simulink model "Mmc"  (R2024b)
settings: Solver=ode23t  StartTime=0.0  StopTime=2  FixedStep=Ts_Power
values from neighbouring files (symbols this model uses):
  C_PM = 10e-3    (= 0.01)    [MmcParameters.m]
  eta = delta_wmax*(Vmax^2)/P_rated    (= 3.64590094798)    [MmcParameters.m]
  Fnom = 50    [MmcParameters.m]
  fs = 1000    [MmcParameters.m]
  I_b = Snom/Vnom_AC/sqrt(3)    [MmcParameters.m]
  Ipp_b = Snom/Vnom_AC/sqrt(3/2)    [MmcParameters.m]
  kicir = R0*alpha_ic    (= 523.598775598)    [MmcParameters.m]
  kpcir = L0*alpha_ic    (= 400)    [MmcParameters.m]
  L0 = 1.2 * L_b    (= 0.0763943726841)    [MmcParameters.m]
  mu = 2*eta*Q_rated/(N*((2*Vmax^2-V0^2)^2-V0^4))    [MmcParameters.m]
  Nb_PM = 20    [MmcParameters.m]
  phi_r = pi/2    (= 1.57079632679)    [MmcParameters.m]
  R0 = .1    (= 0.1)    [MmcParameters.m]
  SCR = 10    [MmcParameters.m]
  SigmaM = 10    [MmcParameters.m]
  Snom = 80e6    (= 80000000)    [MmcParameters.m]
  Ts_Power = 1e-5    (= 1e-05)    [MmcParameters.m]
  V0 = 1    [MmcParameters.m]
  V_b = Vnom_AC    (= 40000)    [MmcParameters.m]
  VDCm = 48e3    (= 48000)    [MmcParameters.m]
  VDCp = 48e3    (= 48000)    [MmcParameters.m]
  Vnom_AC = 40e3    (= 40000)    [MmcParameters.m]
  Vnom_PM = 4.8e3    (= 4800)    [MmcParameters.m]
  w_b = 2*pi*Fnom    (= 314.159265359)    [MmcParameters.m]
  Zn = Vnom_AC^2 / Snom    (= 20)    [MmcParameters.m]
undefined symbols (not defined in the file or in its folder): DiscIntNeverNeededParam
libraries: spsCurrentMeasurementLib x7, spsFirstOrderFilterLib x6, spsHalfBridgeMMCLib x6, spsSeriesRLCBranchLib x6, eePwmGeneratorMultilevel x6, spsVoltageMeasurementLib x4, spsGroundLib x2, spsMeanLib x2, spsDCVoltageSourceLib x2, spsThreePhaseVIMeasurementLib x2, slpidlib x2, spsThreePhaseSeriesRLCLoadLib x2
(part 2 of 3)

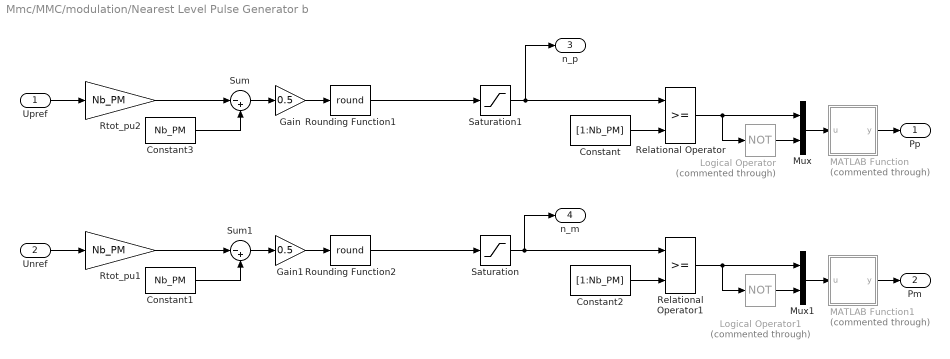
== system Mmc/MMC/modulation/Nearest Level Pulse Generator b ==
  Upref : Inport
  Unref : Inport  Port=2
  Constant : Constant  Value=[1:Nb_PM]
  Constant1 : Constant  Value=Nb_PM
  Constant2 : Constant  Value=[1:Nb_PM]
  Constant3 : Constant  Value=Nb_PM
  Gain : Gain  Gain=0.5
  Gain1 : Gain  Gain=0.5
  Logical Operator : Logic  Commented=through  Operator=NOT  AllPortsSameDT=off  OutDataTypeStr=float('double')
  Logical Operator1 : Logic  Commented=through  Operator=NOT  AllPortsSameDT=off  OutDataTypeStr=float('double')
  MATLAB Function : MATLAB Function  Commented=through  TreatAsAtomicUnit=on
  MATLAB Function1 : MATLAB Function  Commented=through  TreatAsAtomicUnit=on
  Mux : Mux  Inputs=2
  Mux1 : Mux  Inputs=2
  Relational Operator : RelationalOperator  OutDataTypeStr=float('double')  InputSameDT=off
  Relational Operator1 : RelationalOperator  OutDataTypeStr=float('double')  InputSameDT=off
  Rounding Function1 : Rounding  Operator=round
  Rounding Function2 : Rounding  Operator=round
  Rtot_pu1 : Gain  Gain=Nb_PM  SaturateOnIntegerOverflow=on  OutDataTypeStr=Inherit: Same as input  ParamDataTypeStr=Inherit: Same as input
  Rtot_pu2 : Gain  Gain=Nb_PM  SaturateOnIntegerOverflow=on  OutDataTypeStr=Inherit: Same as input  ParamDataTypeStr=Inherit: Same as input
  Saturation : Saturate  UpperLimit=Nb_PM  LowerLimit=0
  Saturation1 : Saturate  UpperLimit=Nb_PM  LowerLimit=0
  Sum : Sum  Inputs=|-+
  Sum1 : Sum  Inputs=|-+
  Pp : Outport  VectorParamsAs1DForOutWhenUnconnected=off
  Pm : Outport  Port=2  VectorParamsAs1DForOutWhenUnconnected=off
  n_p : Outport  Port=3  VectorParamsAs1DForOutWhenUnconnected=off
  n_m : Outport  Port=4  VectorParamsAs1DForOutWhenUnconnected=off
  wires:
  Gain1/1 -> Rounding Function2/1
  Constant1/1 -> Sum1/2
  Rtot_pu1/1 -> Sum1/1
  Unref/1 -> Rtot_pu1/1
  Sum1/1 -> Gain1/1
  Rounding Function2/1 -> Saturation/1
  Rounding Function1/1 -> Saturation1/1
  Saturation/1 -> Relational Operator1/1, n_m/1
  MATLAB Function1/1(y) -> Pm/1
  Mux1/1 -> MATLAB Function1/1(u)
  Logical Operator1/1 -> Mux1/2
  Relational Operator1/1 -> Logical Operator1/1, Mux1/1
  Constant2/1 -> Relational Operator1/2
  Upref/1 -> Rtot_pu2/1
  Gain/1 -> Rounding Function1/1
  Sum/1 -> Gain/1
  Constant3/1 -> Sum/2
  Rtot_pu2/1 -> Sum/1
  Saturation1/1 -> Relational Operator/1, n_p/1
  MATLAB Function/1(y) -> Pp/1
  Mux/1 -> MATLAB Function/1(u)
  Logical Operator/1 -> Mux/2
  Relational Operator/1 -> Mux/1, Logical Operator/1
  Constant/1 -> Relational Operator/2

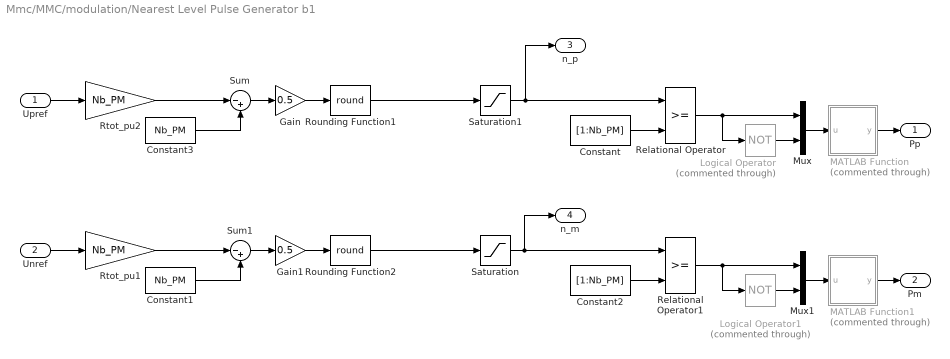
== system Mmc/MMC/modulation/Nearest Level Pulse Generator b1 ==
  Upref : Inport
  Unref : Inport  Port=2
  Constant : Constant  Value=[1:Nb_PM]
  Constant1 : Constant  Value=Nb_PM
  Constant2 : Constant  Value=[1:Nb_PM]
  Constant3 : Constant  Value=Nb_PM
  Gain : Gain  Gain=0.5
  Gain1 : Gain  Gain=0.5
  Logical Operator : Logic  Commented=through  Operator=NOT  AllPortsSameDT=off  OutDataTypeStr=float('double')
  Logical Operator1 : Logic  Commented=through  Operator=NOT  AllPortsSameDT=off  OutDataTypeStr=float('double')
  MATLAB Function : MATLAB Function  Commented=through  TreatAsAtomicUnit=on
  MATLAB Function1 : MATLAB Function  Commented=through  TreatAsAtomicUnit=on
  Mux : Mux  Inputs=2
  Mux1 : Mux  Inputs=2
  Relational Operator : RelationalOperator  OutDataTypeStr=float('double')  InputSameDT=off
  Relational Operator1 : RelationalOperator  OutDataTypeStr=float('double')  InputSameDT=off
  Rounding Function1 : Rounding  Operator=round
  Rounding Function2 : Rounding  Operator=round
  Rtot_pu1 : Gain  Gain=Nb_PM  SaturateOnIntegerOverflow=on  OutDataTypeStr=Inherit: Same as input  ParamDataTypeStr=Inherit: Same as input
  Rtot_pu2 : Gain  Gain=Nb_PM  SaturateOnIntegerOverflow=on  OutDataTypeStr=Inherit: Same as input  ParamDataTypeStr=Inherit: Same as input
  Saturation : Saturate  UpperLimit=Nb_PM  LowerLimit=0
  Saturation1 : Saturate  UpperLimit=Nb_PM  LowerLimit=0
  Sum : Sum  Inputs=|-+
  Sum1 : Sum  Inputs=|-+
  Pp : Outport  VectorParamsAs1DForOutWhenUnconnected=off
  Pm : Outport  Port=2  VectorParamsAs1DForOutWhenUnconnected=off
  n_p : Outport  Port=3  VectorParamsAs1DForOutWhenUnconnected=off
  n_m : Outport  Port=4  VectorParamsAs1DForOutWhenUnconnected=off
  wires:
  Gain1/1 -> Rounding Function2/1
  Constant1/1 -> Sum1/2
  Rtot_pu1/1 -> Sum1/1
  Unref/1 -> Rtot_pu1/1
  Sum1/1 -> Gain1/1
  Rounding Function2/1 -> Saturation/1
  Rounding Function1/1 -> Saturation1/1
  Saturation/1 -> Relational Operator1/1, n_m/1
  MATLAB Function1/1(y) -> Pm/1
  Mux1/1 -> MATLAB Function1/1(u)
  Logical Operator1/1 -> Mux1/2
  Relational Operator1/1 -> Logical Operator1/1, Mux1/1
  Constant2/1 -> Relational Operator1/2
  Upref/1 -> Rtot_pu2/1
  Gain/1 -> Rounding Function1/1
  Sum/1 -> Gain/1
  Constant3/1 -> Sum/2
  Rtot_pu2/1 -> Sum/1
  Saturation1/1 -> Relational Operator/1, n_p/1
  MATLAB Function/1(y) -> Pp/1
  Mux/1 -> MATLAB Function/1(u)
  Logical Operator/1 -> Mux/2
  Relational Operator/1 -> Mux/1, Logical Operator/1
  Constant/1 -> Relational Operator/2

== system Mmc/MMC/modulation/Sorting na ==
  note: A secrect, unintelligible, confusing and insrutable function with \if inside \for inside \if inside \if inside \if
  Usm : Inport
  N : Inport  Port=2
  Iarm : Inport  Port=3
  Constant : Constant  Value=SigmaM
  Logical Operator : Logic  Operator=NOT  AllPortsSameDT=off  OutDataTypeStr=float('double')
  MATLAB Function : MATLAB Function  TreatAsAtomicUnit=on
  MATLAB Function1 : MATLAB Function  TreatAsAtomicUnit=on
  Memory : Memory  InitialCondition=logical(zeros(Nb_PM, 1))  InheritSampleTime=on
  Mux : Mux  Inputs=2
  firing : Outport
  wires:
  MATLAB Function1/1(y) -> firing/1
  Logical Operator/1 -> Mux/2
  MATLAB Function/1(Ons_next) -> Mux/1, Logical Operator/1, Memory/1
  Mux/1 -> MATLAB Function1/1(u)
  Usm/1 -> MATLAB Function/1(Usm)
  Constant/1 -> MATLAB Function/3(Sigmam)
  N/1 -> MATLAB Function/2(N)
  Memory/1 -> MATLAB Function/5(Ons)
  Iarm/1 -> MATLAB Function/4(Iarm)

== system Mmc/MMC/modulation/Sorting nb ==
  note: A secrect, unintelligible, confusing and insrutable function with \if inside \for inside \if inside \if inside \if
  Usm : Inport
  N : Inport  Port=2
  Iarm : Inport  Port=3
  Constant : Constant  Value=SigmaM
  Logical Operator : Logic  Operator=NOT  AllPortsSameDT=off  OutDataTypeStr=float('double')
  MATLAB Function : MATLAB Function  TreatAsAtomicUnit=on
  MATLAB Function1 : MATLAB Function  TreatAsAtomicUnit=on
  Memory : Memory  InitialCondition=logical(zeros(Nb_PM, 1))  InheritSampleTime=on
  Mux : Mux  Inputs=2
  firing : Outport
  wires:
  MATLAB Function1/1(y) -> firing/1
  Logical Operator/1 -> Mux/2
  MATLAB Function/1(Ons_next) -> Mux/1, Logical Operator/1, Memory/1
  Mux/1 -> MATLAB Function1/1(u)
  Usm/1 -> MATLAB Function/1(Usm)
  Constant/1 -> MATLAB Function/3(Sigmam)
  N/1 -> MATLAB Function/2(N)
  Memory/1 -> MATLAB Function/5(Ons)
  Iarm/1 -> MATLAB Function/4(Iarm)

== system Mmc/MMC/modulation/Sorting nc ==
  note: A secrect, unintelligible, confusing and insrutable function with \if inside \for inside \if inside \if inside \if
  Usm : Inport
  N : Inport  Port=2
  Iarm : Inport  Port=3
  Constant : Constant  Value=SigmaM
  Logical Operator : Logic  Operator=NOT  AllPortsSameDT=off  OutDataTypeStr=float('double')
  MATLAB Function : MATLAB Function  TreatAsAtomicUnit=on
  MATLAB Function1 : MATLAB Function  TreatAsAtomicUnit=on
  Memory : Memory  InitialCondition=logical(zeros(Nb_PM, 1))  InheritSampleTime=on
  Mux : Mux  Inputs=2
  firing : Outport
  wires:
  MATLAB Function1/1(y) -> firing/1
  Logical Operator/1 -> Mux/2
  MATLAB Function/1(Ons_next) -> Mux/1, Logical Operator/1, Memory/1
  Mux/1 -> MATLAB Function1/1(u)
  Usm/1 -> MATLAB Function/1(Usm)
  Constant/1 -> MATLAB Function/3(Sigmam)
  N/1 -> MATLAB Function/2(N)
  Memory/1 -> MATLAB Function/5(Ons)
  Iarm/1 -> MATLAB Function/4(Iarm)

== system Mmc/MMC/modulation/Sorting pa ==
  note: A secrect, unintelligible, confusing and insrutable function with \if inside \for inside \if inside \if inside \if
  Usm : Inport
  N : Inport  Port=2
  Iarm : Inport  Port=3
  Constant : Constant  Value=SigmaM
  Logical Operator : Logic  Operator=NOT  AllPortsSameDT=off  OutDataTypeStr=float('double')
  MATLAB Function : MATLAB Function  TreatAsAtomicUnit=on
  MATLAB Function1 : MATLAB Function  TreatAsAtomicUnit=on
  Memory : Memory  InitialCondition=logical(zeros(Nb_PM, 1))  InheritSampleTime=on
  Mux : Mux  Inputs=2
  firing : Outport
  wires:
  Iarm/1 -> MATLAB Function/4(Iarm)
  Memory/1 -> MATLAB Function/5(Ons)
  N/1 -> MATLAB Function/2(N)
  Constant/1 -> MATLAB Function/3(Sigmam)
  Usm/1 -> MATLAB Function/1(Usm)
  Mux/1 -> MATLAB Function1/1(u)
  MATLAB Function/1(Ons_next) -> Memory/1, Logical Operator/1, Mux/1
  Logical Operator/1 -> Mux/2
  MATLAB Function1/1(y) -> firing/1

== system Mmc/MMC/modulation/Sorting pb ==
  note: A secrect, unintelligible, confusing and insrutable function with \if inside \for inside \if inside \if inside \if
  Usm : Inport
  N : Inport  Port=2
  Iarm : Inport  Port=3
  Constant : Constant  Value=SigmaM
  Logical Operator : Logic  Operator=NOT  AllPortsSameDT=off  OutDataTypeStr=float('double')
  MATLAB Function : MATLAB Function  TreatAsAtomicUnit=on
  MATLAB Function1 : MATLAB Function  TreatAsAtomicUnit=on
  Memory : Memory  InitialCondition=logical(zeros(Nb_PM, 1))  InheritSampleTime=on
  Mux : Mux  Inputs=2
  firing : Outport
  wires:
  Iarm/1 -> MATLAB Function/4(Iarm)
  Memory/1 -> MATLAB Function/5(Ons)
  N/1 -> MATLAB Function/2(N)
  Constant/1 -> MATLAB Function/3(Sigmam)
  Usm/1 -> MATLAB Function/1(Usm)
  Mux/1 -> MATLAB Function1/1(u)
  MATLAB Function/1(Ons_next) -> Memory/1, Logical Operator/1, Mux/1
  Logical Operator/1 -> Mux/2
  MATLAB Function1/1(y) -> firing/1

== system Mmc/MMC/modulation/Sorting pc ==
  note: A secrect, unintelligible, confusing and insrutable function with \if inside \for inside \if inside \if inside \if
  Usm : Inport
  N : Inport  Port=2
  Iarm : Inport  Port=3
  Constant : Constant  Value=SigmaM
  Logical Operator : Logic  Operator=NOT  AllPortsSameDT=off  OutDataTypeStr=float('double')
  MATLAB Function : MATLAB Function  TreatAsAtomicUnit=on
  MATLAB Function1 : MATLAB Function  TreatAsAtomicUnit=on
  Memory : Memory  InitialCondition=logical(zeros(Nb_PM, 1))  InheritSampleTime=on
  Mux : Mux  Inputs=2
  firing : Outport
  wires:
  Iarm/1 -> MATLAB Function/4(Iarm)
  Memory/1 -> MATLAB Function/5(Ons)
  N/1 -> MATLAB Function/2(N)
  Constant/1 -> MATLAB Function/3(Sigmam)
  Usm/1 -> MATLAB Function/1(Usm)
  Mux/1 -> MATLAB Function1/1(u)
  MATLAB Function/1(Ons_next) -> Memory/1, Logical Operator/1, Mux/1
  Logical Operator/1 -> Mux/2
  MATLAB Function1/1(y) -> firing/1

== system Mmc/MMC/modulation/Subsystem10 ==
  ref : Inport
  PWM Generator (Multilevel) : eePwmGeneratorMultilevel/PWM Generator (Multilevel)  topology=Half-bridge  Nsm=20  Tper=1/fs  Ts=Ts_Power
  Scope : Scope
  Upper arm a : MATLAB Function  TreatAsAtomicUnit=on
  n_pwm : Outport
  wires:
  ref/1 -> PWM Generator (Multilevel)/1
  Upper arm a/1(n_pwm) -> n_pwm/1, Scope/1
  PWM Generator (Multilevel)/1 -> Upper arm a/1(signals)

== system Mmc/MMC/modulation/Subsystem11 ==
  ref : Inport
  PWM Generator (Multilevel) : eePwmGeneratorMultilevel/PWM Generator (Multilevel)  topology=Half-bridge  Nsm=20  Tper=1/fs  Ts=Ts_Power
  Scope : Scope
  Upper arm a : MATLAB Function  TreatAsAtomicUnit=on
  n_pwm : Outport
  wires:
  PWM Generator (Multilevel)/1 -> Upper arm a/1(signals)
  Upper arm a/1(n_pwm) -> Scope/1, n_pwm/1
  ref/1 -> PWM Generator (Multilevel)/1

== system Mmc/MMC/modulation/Subsystem6 ==
  ref : Inport
  PWM Generator (Multilevel) : eePwmGeneratorMultilevel/PWM Generator (Multilevel)  topology=Half-bridge  Nsm=20  Tper=1/fs  Ts=Ts_Power
  Scope : Scope
  Upper arm a : MATLAB Function  TreatAsAtomicUnit=on
  n_pwm : Outport
  wires:
  ref/1 -> PWM Generator (Multilevel)/1
  Upper arm a/1(n_pwm) -> n_pwm/1, Scope/1
  PWM Generator (Multilevel)/1 -> Upper arm a/1(signals)

== system Mmc/MMC/modulation/Subsystem7 ==
  ref : Inport
  PWM Generator (Multilevel) : eePwmGeneratorMultilevel/PWM Generator (Multilevel)  topology=Half-bridge  Nsm=20  Tper=1/fs  Ts=Ts_Power
  Scope : Scope
  Upper arm a : MATLAB Function  TreatAsAtomicUnit=on
  n_pwm : Outport
  wires:
  PWM Generator (Multilevel)/1 -> Upper arm a/1(signals)
  Upper arm a/1(n_pwm) -> Scope/1, n_pwm/1
  ref/1 -> PWM Generator (Multilevel)/1

== system Mmc/MMC/modulation/Subsystem8 ==
  ref : Inport
  PWM Generator (Multilevel) : eePwmGeneratorMultilevel/PWM Generator (Multilevel)  topology=Half-bridge  Nsm=20  Tper=1/fs  Ts=Ts_Power
  Scope : Scope
  Upper arm a : MATLAB Function  TreatAsAtomicUnit=on
  n_pwm : Outport
  wires:
  ref/1 -> PWM Generator (Multilevel)/1
  Upper arm a/1(n_pwm) -> n_pwm/1, Scope/1
  PWM Generator (Multilevel)/1 -> Upper arm a/1(signals)

== system Mmc/MMC/modulation/Subsystem9 ==
  ref : Inport
  PWM Generator (Multilevel) : eePwmGeneratorMultilevel/PWM Generator (Multilevel)  topology=Half-bridge  Nsm=20  Tper=1/fs  Ts=Ts_Power
  Scope : Scope
  Upper arm a : MATLAB Function  TreatAsAtomicUnit=on
  n_pwm : Outport
  wires:
  PWM Generator (Multilevel)/1 -> Upper arm a/1(signals)
  Upper arm a/1(n_pwm) -> Scope/1, n_pwm/1
  ref/1 -> PWM Generator (Multilevel)/1

== system Mmc/MMC/reference voltage generator/dq0 to abc1 ==
  dq0 : Inport
  theta : Inport  Port=2
  Add : Sum
  Demux : Demux  Outputs=3
  Gain : Gain  Gain=1/2
  Gain1 : Gain  Gain=sqrt(3)/2
  Mux : Mux  Inputs=3
  Product{,1..3} (4 alike) : Product
  Subtract : Sum  Inputs=+-
  Subtract1 : Sum
  Subtract2 : Sum  Inputs=-++
  Subtract3 : Sum  Inputs=--+
  Trigonometric Function : Trigonometry
  Trigonometric Function1 : Trigonometry  Operator=cos
  abc : Outport
  wires:
  theta/1 -> Trigonometric Function1/1, Trigonometric Function/1
  Demux/1 -> Product3/1, Product1/1
  Demux/2 -> Product2/1, Product/1
  Trigonometric Function/1 -> Product1/2, Product2/2
  Trigonometric Function1/1 -> Product/2, Product3/2
  Product3/1 -> Subtract/1
  Product1/1 -> Subtract1/1
  Product/1 -> Subtract1/2
  Product2/1 -> Subtract/2
  Subtract/1 -> Add/1, Gain/1
  Subtract1/1 -> Gain1/1
  Gain/1 -> Subtract3/1, Subtract2/1
  Gain1/1 -> Subtract2/2, Subtract3/2
  Subtract3/1 -> Mux/3
  Subtract2/1 -> Mux/2
  Mux/1 -> abc/1
  dq0/1 -> Demux/1
  Demux/3 -> Subtract2/3, Subtract3/3, Add/2
  Add/1 -> Mux/1

== system Mmc/MMC/reference voltage generator/dq0 to abc2 ==
  dq0 : Inport
  theta : Inport  Port=2
  Add : Sum
  Demux : Demux  Outputs=3
  Gain : Gain  Gain=1/2
  Gain1 : Gain  Gain=sqrt(3)/2
  Mux : Mux  Inputs=3
  Product{,1..3} (4 alike) : Product
  Subtract : Sum  Inputs=+-
  Subtract1 : Sum
  Subtract2 : Sum  Inputs=-++
  Subtract3 : Sum  Inputs=--+
  Trigonometric Function : Trigonometry
  Trigonometric Function1 : Trigonometry  Operator=cos
  abc : Outport
  wires:
  theta/1 -> Trigonometric Function1/1, Trigonometric Function/1
  Demux/1 -> Product3/1, Product1/1
  Demux/2 -> Product2/1, Product/1
  Trigonometric Function/1 -> Product1/2, Product2/2
  Trigonometric Function1/1 -> Product/2, Product3/2
  Product3/1 -> Subtract/1
  Product1/1 -> Subtract1/1
  Product/1 -> Subtract1/2
  Product2/1 -> Subtract/2
  Subtract/1 -> Add/1, Gain/1
  Subtract1/1 -> Gain1/1
  Gain/1 -> Subtract3/1, Subtract2/1
  Gain1/1 -> Subtract2/2, Subtract3/2
  Subtract3/1 -> Mux/3
  Subtract2/1 -> Mux/2
  Mux/1 -> abc/1
  dq0/1 -> Demux/1
  Demux/3 -> Subtract2/3, Subtract3/3, Add/2
  Add/1 -> Mux/1

== system Mmc/MMC/uVOC/abc to alpha beta ==
  abc : Inport
  Demux : Demux  Outputs=3
  Gain : Gain  Gain=2/3
  Gain1 : Gain  Gain=1/2
  Gain2 : Gain  Gain=sqrt(3)/2
  Gain3 : Gain  Gain=0
  Gain4 : Gain  Gain=1/2
  Gain5 : Gain  Gain=1/2
  Gain6 : Gain  Gain=sqrt(3)/2
  Mux : Mux  Inputs=3
  Subtract : Sum  Inputs=+--
  Subtract1 : Sum  Inputs=++-
  Subtract2 : Sum  Inputs=+++
  alpha beta 0 : Outport
  wires:
  abc/1 -> Demux/1
  Mux/1 -> Gain/1
  Gain/1 -> alpha beta 0/1
  Subtract/1 -> Mux/1
  Subtract1/1 -> Mux/2
  Subtract2/1 -> Mux/3
  Demux/1 -> Gain1/1, Gain3/1, Subtract/1
  Gain3/1 -> Subtract1/1
  Gain1/1 -> Subtract2/1
  Demux/2 -> Gain2/1, Gain4/1
  Gain4/1 -> Subtract2/2, Subtract/2
  Gain2/1 -> Subtract1/2
  Demux/3 -> Gain6/1, Gain5/1
  Gain5/1 -> Subtract2/3, Subtract/3
  Gain6/1 -> Subtract1/3

== system Mmc/MMC/uVOC/abc to alpha beta1 ==
  abc : Inport
  Demux : Demux  Outputs=3
  Gain : Gain  Gain=2/3
  Gain1 : Gain  Gain=1/2
  Gain2 : Gain  Gain=sqrt(3)/2
  Gain3 : Gain  Gain=0
  Gain4 : Gain  Gain=1/2
  Gain5 : Gain  Gain=1/2
  Gain6 : Gain  Gain=sqrt(3)/2
  Mux : Mux  Inputs=3
  Subtract : Sum  Inputs=+--
  Subtract1 : Sum  Inputs=++-
  Subtract2 : Sum  Inputs=+++
  alpha beta 0 : Outport
  wires:
  abc/1 -> Demux/1
  Mux/1 -> Gain/1
  Gain/1 -> alpha beta 0/1
  Subtract/1 -> Mux/1
  Subtract1/1 -> Mux/2
  Subtract2/1 -> Mux/3
  Demux/1 -> Gain1/1, Gain3/1, Subtract/1
  Gain3/1 -> Subtract1/1
  Gain1/1 -> Subtract2/1
  Demux/2 -> Gain2/1, Gain4/1
  Gain4/1 -> Subtract2/2, Subtract/2
  Gain2/1 -> Subtract1/2
  Demux/3 -> Gain6/1, Gain5/1
  Gain5/1 -> Subtract2/3, Subtract/3
  Gain6/1 -> Subtract1/3

== system Mmc/MMC/uVOC/abc to alpha beta2 ==
  abc : Inport
  Demux : Demux  Outputs=3
  Gain : Gain  Gain=2/3
  Gain1 : Gain  Gain=1/2
  Gain2 : Gain  Gain=sqrt(3)/2
  Gain3 : Gain  Gain=0
  Gain4 : Gain  Gain=1/2
  Gain5 : Gain  Gain=1/2
  Gain6 : Gain  Gain=sqrt(3)/2
  Mux : Mux  Inputs=3
  Subtract : Sum  Inputs=+--
  Subtract1 : Sum  Inputs=++-
  Subtract2 : Sum  Inputs=+++
  alpha beta 0 : Outport
  wires:
  abc/1 -> Demux/1
  Mux/1 -> Gain/1
  Gain/1 -> alpha beta 0/1
  Subtract/1 -> Mux/1
  Subtract1/1 -> Mux/2
  Subtract2/1 -> Mux/3
  Demux/1 -> Gain1/1, Gain3/1, Subtract/1
  Gain3/1 -> Subtract1/1
  Gain1/1 -> Subtract2/1
  Demux/2 -> Gain2/1, Gain4/1
  Gain4/1 -> Subtract2/2, Subtract/2
  Gain2/1 -> Subtract1/2
  Demux/3 -> Gain6/1, Gain5/1
  Gain5/1 -> Subtract2/3, Subtract/3
  Gain6/1 -> Subtract1/3

== system Mmc/MMC/uVOC/abc to dq ==
  abc : Inport
  theta : Inport  Port=2
  Demux : Demux  Outputs=3
  Gain : Gain  Gain=2/3
  Gain1 : Gain  Gain=1/3
  Gain2 : Gain  Gain=1/sqrt(3)
  Mux : Mux  Inputs=2
  Product{,1..3} (4 alike) : Product
  Subtract : Sum
  Subtract1 : Sum  Inputs=+-
  Subtract2 : Sum  Inputs=+-
  Subtract3 : Sum
  Subtract4 : Sum  Inputs=-+
  Trigonometric Function : Trigonometry
  Trigonometric Function1 : Trigonometry  Operator=cos
  dq : Outport
  wires:
  abc/1 -> Demux/1
  Demux/1 -> Gain/1
  Demux/3 -> Subtract1/2, Subtract/2
  Demux/2 -> Subtract1/1, Subtract/1
  Subtract/1 -> Gain1/1
  Subtract1/1 -> Gain2/1
  Gain/1 -> Subtract2/1
  Gain1/1 -> Subtract2/2
  Subtract2/1 -> Product2/1, Product/1
  Product/1 -> Subtract3/1
  Product1/1 -> Subtract3/2
  Product2/1 -> Subtract4/1
  Product3/1 -> Subtract4/2
  Mux/1 -> dq/1
  Subtract3/1 -> Mux/1
  Subtract4/1 -> Mux/2
  theta/1 -> Trigonometric Function/1, Trigonometric Function1/1
  Trigonometric Function/1 -> Product2/2, Product1/2
  Trigonometric Function1/1 -> Product/2, Product3/2
  Gain2/1 -> Product1/1

== system Mmc/MMC/uVOC/abc to dq0 ==
  abc : Inport
  theta : Inport  Port=2
  Demux : Demux  Outputs=3
  Gain : Gain  Gain=2/3
  Gain1 : Gain  Gain=1/3
  Gain2 : Gain  Gain=1/sqrt(3)
  Gain3 : Gain  Gain=1/2
  Gain4 : Gain  Gain=1/2
  Gain5 : Gain  Gain=1/2
  Mux : Mux  Inputs=3
  Product{,1..3} (4 alike) : Product
  Subtract : Sum
  Subtract1 : Sum  Inputs=+-
  Subtract2 : Sum  Inputs=+-
  Subtract3 : Sum
  Subtract4 : Sum  Inputs=-+
  Subtract5 : Sum  Inputs=+++
  Trigonometric Function : Trigonometry
  Trigonometric Function1 : Trigonometry  Operator=cos
  dq0 : Outport
  wires:
  abc/1 -> Demux/1
  Demux/1 -> Gain3/1, Gain/1
  Demux/3 -> Gain5/1, Subtract1/2, Subtract/2
  Demux/2 -> Subtract/1, Subtract1/1, Gain4/1
  Subtract/1 -> Gain1/1
  Subtract1/1 -> Gain2/1
  Gain/1 -> Subtract2/1
  Gain1/1 -> Subtract2/2
  Subtract2/1 -> Product2/1, Product/1
  Product/1 -> Subtract3/1
  Product1/1 -> Subtract3/2
  Product2/1 -> Subtract4/1
  Product3/1 -> Subtract4/2
  Mux/1 -> dq0/1
  Subtract3/1 -> Mux/1
  Subtract4/1 -> Mux/2
  theta/1 -> Trigonometric Function/1, Trigonometric Function1/1
  Trigonometric Function/1 -> Product2/2, Product1/2
  Trigonometric Function1/1 -> Product/2, Product3/2
  Gain2/1 -> Product1/1
  Subtract5/1 -> Mux/3
  Gain3/1 -> Subtract5/1
  Gain4/1 -> Subtract5/2
  Gain5/1 -> Subtract5/3

== system Mmc/MMC/uVOC/alpha beta dq ==
  alpha beta 0 : Inport
  theta : Inport  Port=2
  Add1 : Sum
  Add2 : Sum  Inputs=-+
  Constant : Constant  Value=0
  Demux : Demux  Outputs=3
  Mux : Mux  Inputs=3
  Product{,1..3} (4 alike) : Product
  Terminator : Terminator
  Trigonometric Function : Trigonometry
  Trigonometric Function1 : Trigonometry  Operator=cos
  dq0 : Outport
  wires:
  alpha beta 0/1 -> Demux/1
  Demux/3 -> Terminator/1
  Mux/1 -> dq0/1
  theta/1 -> Trigonometric Function1/1, Trigonometric Function/1
  Add1/1 -> Mux/1
  Add2/1 -> Mux/2
  Trigonometric Function/1 -> Product1/1, Product2/1
  Demux/1 -> Product/2, Product2/2
  Trigonometric Function1/1 -> Product3/1, Product/1
  Demux/2 -> Product3/2, Product1/2
  Product/1 -> Add1/1
  Product1/1 -> Add1/2
  Product2/1 -> Add2/1
  Product3/1 -> Add2/2
  Constant/1 -> Mux/3

== system Mmc/MMC/uVOC/alpha beta dq1 ==
  alpha beta 0 : Inport
  theta : Inport  Port=2
  Add1 : Sum
  Add2 : Sum  Inputs=-+
  Constant : Constant  Value=0
  Demux : Demux  Outputs=3
  Mux : Mux  Inputs=3
  Product{,1..3} (4 alike) : Product
  Terminator : Terminator
  Trigonometric Function : Trigonometry
  Trigonometric Function1 : Trigonometry  Operator=cos
  dq0 : Outport
  wires:
  alpha beta 0/1 -> Demux/1
  Demux/3 -> Terminator/1
  Mux/1 -> dq0/1
  theta/1 -> Trigonometric Function1/1, Trigonometric Function/1
  Add1/1 -> Mux/1
  Add2/1 -> Mux/2
  Trigonometric Function/1 -> Product1/1, Product2/1
  Demux/1 -> Product/2, Product2/2
  Trigonometric Function1/1 -> Product3/1, Product/1
  Demux/2 -> Product3/2, Product1/2
  Product/1 -> Add1/1
  Product1/1 -> Add1/2
  Product2/1 -> Add2/1
  Product3/1 -> Add2/2
  Constant/1 -> Mux/3

== system Mmc/MMC/uVOC/alpha beta to abc ==
  alpha beta 0 : Inport
  Demux : Demux  Outputs=3
  Gain : Gain
  Gain1 : Gain  Gain=1/2
  Gain2 : Gain  Gain=sqrt(3)/2
  Gain3 : Gain  Gain=0
  Mux : Mux  Inputs=3
  Subtract : Sum  Inputs=+++
  Subtract1 : Sum  Inputs=-++
  Subtract2 : Sum  Inputs=--+
  abc : Outport
  wires:
  alpha beta 0/1 -> Demux/1
  Mux/1 -> Gain/1
  Gain/1 -> abc/1
  Subtract/1 -> Mux/1
  Subtract1/1 -> Mux/2
  Subtract2/1 -> Mux/3
  Demux/1 -> Gain1/1, Subtract/1
  Gain1/1 -> Subtract2/1, Subtract1/1
  Demux/2 -> Gain3/1, Gain2/1
  Gain2/1 -> Subtract2/2, Subtract1/2
  Gain3/1 -> Subtract/2
  Demux/3 -> Subtract2/3, Subtract1/3, Subtract/3

== system Mmc/MMC/uVOC/alpha beta to abc1 ==
  alpha beta 0 : Inport
  Demux : Demux  Outputs=3
  Gain : Gain
  Gain1 : Gain  Gain=1/2
  Gain2 : Gain  Gain=sqrt(3)/2
  Gain3 : Gain  Gain=0
  Mux : Mux  Inputs=3
  Subtract : Sum  Inputs=+++
  Subtract1 : Sum  Inputs=-++
  Subtract2 : Sum  Inputs=--+
  abc : Outport
  wires:
  alpha beta 0/1 -> Demux/1
  Mux/1 -> Gain/1
  Gain/1 -> abc/1
  Subtract/1 -> Mux/1
  Subtract1/1 -> Mux/2
  Subtract2/1 -> Mux/3
  Demux/1 -> Gain1/1, Subtract/1
  Gain1/1 -> Subtract2/1, Subtract1/1
  Demux/2 -> Gain3/1, Gain2/1
  Gain2/1 -> Subtract2/2, Subtract1/2
  Gain3/1 -> Subtract/2
  Demux/3 -> Subtract2/3, Subtract1/3, Subtract/3

== system Mmc/MMC/uVOC/alpha beta to abc2 ==
  theta : Inport
  alpha beta : Inport  Port=2
  Demux : Demux  Outputs=2
  Gain : Gain  Gain=1/2
  Gain1 : Gain  Gain=sqrt(3)/2
  Mux : Mux  Inputs=3
  Product{,1..3} (4 alike) : Product
  Subtract : Sum  Inputs=+-
  Subtract1 : Sum
  Subtract2 : Sum  Inputs=-+
  Subtract3 : Sum  Inputs=--
  Trigonometric Function : Trigonometry
  Trigonometric Function1 : Trigonometry  Operator=cos
  abc : Outport
  wires:
  theta/1 -> Trigonometric Function1/1, Trigonometric Function/1
  Demux/1 -> Product1/1, Product3/1
  Demux/2 -> Product2/1, Product/1
  Trigonometric Function/1 -> Product1/2, Product2/2
  Trigonometric Function1/1 -> Product/2, Product3/2
  Product3/1 -> Subtract/1
  Product1/1 -> Subtract1/1
  Product/1 -> Subtract1/2
  Product2/1 -> Subtract/2
  Subtract/1 -> Mux/1, Gain/1
  Subtract1/1 -> Gain1/1
  Gain/1 -> Subtract3/1, Subtract2/1
  Gain1/1 -> Subtract2/2, Subtract3/2
  Subtract3/1 -> Mux/3
  Subtract2/1 -> Mux/2
  Mux/1 -> abc/1
  alpha beta/1 -> Demux/1

== system Mmc/MMC/uVOC/dq alpha beta ==
  dq0 : Inport
  theta : Inport  Port=2
  Add1 : Sum  Inputs=+-
  Add2 : Sum
  Constant : Constant  Value=0
  Demux : Demux  Outputs=3
  Mux : Mux  Inputs=3
  Product{,1..3} (4 alike) : Product
  Terminator : Terminator
  Trigonometric Function : Trigonometry
  Trigonometric Function1 : Trigonometry  Operator=cos
  alpha beta 0 : Outport
  wires:
  dq0/1 -> Demux/1
  Demux/3 -> Terminator/1
  Mux/1 -> alpha beta 0/1
  theta/1 -> Trigonometric Function1/1, Trigonometric Function/1
  Add1/1 -> Mux/1
  Add2/1 -> Mux/2
  Trigonometric Function/1 -> Product2/2, Product1/2
  Demux/2 -> Product3/1, Product1/1
  Constant/1 -> Mux/3
  Demux/1 -> Product2/1, Product/1
  Product2/1 -> Add2/1
  Product3/1 -> Add2/2
  Product/1 -> Add1/1
  Product1/1 -> Add1/2
  Trigonometric Function1/1 -> Product3/2, Product/2

== system Mmc/MMC/uVOC/dq to abc ==
  theta : Inport
  dq : Inport  Port=2
  Demux : Demux  Outputs=2
  Gain : Gain  Gain=1/2
  Gain1 : Gain  Gain=sqrt(3)/2
  Mux : Mux  Inputs=3
  Product{,1..3} (4 alike) : Product
  Subtract : Sum  Inputs=+-
  Subtract1 : Sum
  Subtract2 : Sum  Inputs=-+
  Subtract3 : Sum  Inputs=--
  Trigonometric Function : Trigonometry
  Trigonometric Function1 : Trigonometry  Operator=cos
  abc : Outport
  wires:
  theta/1 -> Trigonometric Function1/1, Trigonometric Function/1
  Demux/1 -> Product1/1, Product3/1
  Demux/2 -> Product2/1, Product/1
  Trigonometric Function/1 -> Product1/2, Product2/2
  Trigonometric Function1/1 -> Product/2, Product3/2
  Product3/1 -> Subtract/1
  Product1/1 -> Subtract1/1
  Product/1 -> Subtract1/2
  Product2/1 -> Subtract/2
  Subtract/1 -> Mux/1, Gain/1
  Subtract1/1 -> Gain1/1
  Gain/1 -> Subtract3/1, Subtract2/1
  Gain1/1 -> Subtract2/2, Subtract3/2
  Subtract3/1 -> Mux/3
  Subtract2/1 -> Mux/2
  Mux/1 -> abc/1
  dq/1 -> Demux/1

== system Mmc/MMC/uVOC/dq0 to abc ==
  theta : Inport
  dq0 : Inport  Port=2
  Add : Sum
  Demux : Demux  Outputs=3
  Gain : Gain  Gain=1/2
  Gain1 : Gain  Gain=sqrt(3)/2
  Mux : Mux  Inputs=3
  Product{,1..3} (4 alike) : Product
  Subtract : Sum  Inputs=+-
  Subtract1 : Sum
  Subtract2 : Sum  Inputs=-++
  Subtract3 : Sum  Inputs=--+
  Trigonometric Function : Trigonometry
  Trigonometric Function1 : Trigonometry  Operator=cos
  abc : Outport
  wires:
  theta/1 -> Trigonometric Function1/1, Trigonometric Function/1
  Demux/1 -> Product3/1, Product1/1
  Demux/2 -> Product2/1, Product/1
  Trigonometric Function/1 -> Product1/2, Product2/2
  Trigonometric Function1/1 -> Product/2, Product3/2
  Product3/1 -> Subtract/1
  Product1/1 -> Subtract1/1
  Product/1 -> Subtract1/2
  Product2/1 -> Subtract/2
  Subtract/1 -> Add/1, Gain/1
  Subtract1/1 -> Gain1/1
  Gain/1 -> Subtract3/1, Subtract2/1
  Gain1/1 -> Subtract2/2, Subtract3/2
  Subtract3/1 -> Mux/3
  Subtract2/1 -> Mux/2
  Mux/1 -> abc/1
  dq0/1 -> Demux/1
  Demux/3 -> Subtract2/3, Subtract3/3, Add/2
  Add/1 -> Mux/1

== matlab function Mmc/MMC/modulation/Subsystem9/Upper arm a ==
  data: signals input; n_pwm output
function n_pwm = PWM(signals)
% Name: PWM
% Input: the PWM gate signal of one arm.
%        40 signals with 0 or 1 
% Output: the number of activated submodels in one arm
%         0<Int(n_pwm)<20
% Discription: Get the number of activated submodels from the PWM gate
% signals

    % Identify if there is 40 signal inputs
    if length(signals) ~= 40
        error('Input must be a vector with exactly 40 elements.');
    end
    % Select the odd signal (the gate signal for upper side switch)
    Sig_up = signals(1:2:end);
    % Count how many submodel is activated
    n_pwm = 20 - sum(Sig_up);
end

== matlab function Mmc/MMC/modulation/Nearest Level Pulse Generator a /MATLAB Function1 ==
  data: u input; y output
function y = FiringSorting(u)
    y = u;
    for i = 1: length(u)
        if mod(i, 2) == 1
            y(i) = u(int16(i/2));
        else
            y(i) = u(int16(i/2+length(u)/2));
        end
    end
end

== matlab function Mmc/MMC/modulation/Sorting na/MATLAB Function ==
  data: Usm input; N input; Ons_next output; Sigmam input; Iarm input; Ons input
function Ons_next = SmFiringSorting(Usm, N, Sigmam, Iarm, Ons)
    %%%
    % SmFiringSorting -- SM firing sorting. -- C.SI on 5th, Oct.
    %% Inputs:
    % Usm - capacitor voltage on each SM;
    % N - number of SMs that needed to fire up;
    % Sigmam [%] - Maximum allowed voltage unbalance rate;
    % Iarm - arm current;
    % Ons (boolean) - indicate those SM(s) who are in series with the
    % source in the last control period;
    %% Outputs:
    % Ons_now (boolean) - indicate those SM(s) who should be in series with 
    % the source in this control period;
    %%%
    
    % number of SMs
    Nb = length(Usm);
    % initialize the on-state boolean array
    Ons_next = zeros(Nb, 1); 
    % rank the SMs in the order of descendance
    [~, order] = sort(Usm, 'descend');
    
    if max(abs(1-Usm)) > Sigmam/100
        % Over the maximum unbalance acceptance
        if Iarm > 0
            % charge the capacitors with lowest voltages
            Ons_next(order(Nb-N+1: Nb)) = ~Ons_next(order(Nb-N+1: Nb));
        else
            % discharge the capacitors with highest voltages
            Ons_next(order(1: N)) = ~Ons_next(order(1: N));
        end

    else
        if N-sum(Ons) ==  0
            % if we don't need to change the number of SM that is on
            Ons_next = Ons;
        
        elseif N-sum(Ons) > 0
            % if we need more SMs are to be on-state

            % number of SMs that needed to be changed the state
            DeltaN = N-sum(Ons);
            % keep previously being on SMs still being on
            Ons_next = Ons;

            if Iarm > 0
                % charge the capacitors with lowest voltages
                for i = 1: Nb
                    if DeltaN <= 0
                        break;
                    end
                    % if the SM is off and still need more SM
                    if Ons(order(Nb-i+1)) == false
                        DeltaN = DeltaN - 1;
                        Ons_next(order(Nb-i+1)) = true;
                    end
                end

            else
                % discharge the capacitors with highest voltages
                for i = 1: Nb
                    if DeltaN <= 0
                        break;
                    end
                    % if the SM is off and still need more SM
                    if Ons(order(i)) == false
                        DeltaN = DeltaN - 1;
                        Ons_next(order(i)) = true;
                    end
                end
            end

        else
            % if we need less SMs are to be on-state

            % number of SMs that needed to be changed the state
            DeltaN = sum(Ons)-N;
            % keep previously being on SMs still being on
            Ons_next = Ons;

            if Iarm > 0
                % remove the capacitor with highest voltage
                for i = 1: Nb
                    if DeltaN <= 0
                        break;
                    end
                    % if the SM is on and still need less SM
                    if Ons(order(i)) == true
                        DeltaN = DeltaN - 1;
                        Ons_next(order(i)) = false;
                    end
                end

            else
                % remove the capacitor with lowest voltage
                for i = 1: Nb
                    if DeltaN <= 0
                        break;
                    end
                    % if the SM is on and still need less SM
                    if Ons(order(Nb-i+1)) == true
                        DeltaN = DeltaN - 1;
                        Ons_next(order(Nb-i+1)) = false;
                    end
                end
            end
        end
    end
end

== matlab function Mmc/MMC/modulation/Sorting na/MATLAB Function1 ==
  data: u input; y output
function y = FiringSorting(u)
    y = u;
    for i = 1: length(u)
        if mod(i, 2) == 1
            y(i) = u(int16(i/2));
        else
            y(i) = u(int16(i/2+length(u)/2));
        end
    end
end

== matlab function Mmc/MMC/modulation/Sorting pb/MATLAB Function ==
  data: Usm input; N input; Ons_next output; Sigmam input; Iarm input; Ons input
function Ons_next = SmFiringSorting(Usm, N, Sigmam, Iarm, Ons)
    %%%
    % SmFiringSorting -- SM firing sorting. -- C.SI on 5th, Oct.
    %% Inputs:
    % Usm - capacitor voltage on each SM;
    % N - number of SMs that needed to fire up;
    % Sigmam [%] - Maximum allowed voltage unbalance rate;
    % Iarm - arm current;
    % Ons (boolean) - indicate those SM(s) who are in series with the
    % source in the last control period;
    %% Outputs:
    % Ons_now (boolean) - indicate those SM(s) who should be in series with 
    % the source in this control period;
    %%%
    
    % number of SMs
    Nb = length(Usm);
    % initialize the on-state boolean array
    Ons_next = zeros(Nb, 1); 
    % rank the SMs in the order of descendance
    [~, order] = sort(Usm, 'descend');
    
    if max(abs(1-Usm)) > Sigmam/100
        % Over the maximum unbalance acceptance
        if Iarm > 0
            % charge the capacitors with lowest voltages
            Ons_next(order(Nb-N+1: Nb)) = ~Ons_next(order(Nb-N+1: Nb));
        else
            % discharge the capacitors with highest voltages
            Ons_next(order(1: N)) = ~Ons_next(order(1: N));
        end

    else
        if N-sum(Ons) ==  0
            % if we don't need to change the number of SM that is on
            Ons_next = Ons;
        
        elseif N-sum(Ons) > 0
            % if we need more SMs are to be on-state

            % number of SMs that needed to be changed the state
            DeltaN = N-sum(Ons);
            % keep previously being on SMs still being on
            Ons_next = Ons;

            if Iarm > 0
                % charge the capacitors with lowest voltages
                for i = 1: Nb
                    if DeltaN <= 0
                        break;
                    end
                    % if the SM is off and still need more SM
                    if Ons(order(Nb-i+1)) == false
                        DeltaN = DeltaN - 1;
                        Ons_next(order(Nb-i+1)) = true;
                    end
                end

            else
                % discharge the capacitors with highest voltages
                for i = 1: Nb
                    if DeltaN <= 0
                        break;
                    end
                    % if the SM is off and still need more SM
                    if Ons(order(i)) == false
                        DeltaN = DeltaN - 1;
                        Ons_next(order(i)) = true;
                    end
                end
            end

        else
            % if we need less SMs are to be on-state

            % number of SMs that needed to be changed the state
            DeltaN = sum(Ons)-N;
            % keep previously being on SMs still being on
            Ons_next = Ons;

            if Iarm > 0
                % remove the capacitor with highest voltage
                for i = 1: Nb
                    if DeltaN <= 0
                        break;
                    end
                    % if the SM is on and still need less SM
                    if Ons(order(i)) == true
                        DeltaN = DeltaN - 1;
                        Ons_next(order(i)) = false;
                    end
                end

            else
                % remove the capacitor with lowest voltage
                for i = 1: Nb
                    if DeltaN <= 0
                        break;
                    end
                    % if the SM is on and still need less SM
                    if Ons(order(Nb-i+1)) == true
                        DeltaN = DeltaN - 1;
                        Ons_next(order(Nb-i+1)) = false;
                    end
                end
            end
        end
    end
end

== matlab function Mmc/MMC/modulation/Sorting pb/MATLAB Function1 ==
  data: u input; y output
function y = FiringSorting(u)
    y = u;
    for i = 1: length(u)
        if mod(i, 2) == 1
            y(i) = u(int16(i/2));
        else
            y(i) = u(int16(i/2+length(u)/2));
        end
    end
end

== matlab function Mmc/MMC/modulation/Sorting nb/MATLAB Function ==
  data: Usm input; N input; Ons_next output; Sigmam input; Iarm input; Ons input
function Ons_next = SmFiringSorting(Usm, N, Sigmam, Iarm, Ons)
    %%%
    % SmFiringSorting -- SM firing sorting. -- C.SI on 5th, Oct.
    %% Inputs:
    % Usm - capacitor voltage on each SM;
    % N - number of SMs that needed to fire up;
    % Sigmam [%] - Maximum allowed voltage unbalance rate;
    % Iarm - arm current;
    % Ons (boolean) - indicate those SM(s) who are in series with the
    % source in the last control period;
    %% Outputs:
    % Ons_now (boolean) - indicate those SM(s) who should be in series with 
    % the source in this control period;
    %%%
    
    % number of SMs
    Nb = length(Usm);
    % initialize the on-state boolean array
    Ons_next = zeros(Nb, 1); 
    % rank the SMs in the order of descendance
    [~, order] = sort(Usm, 'descend');
    
    if max(abs(1-Usm)) > Sigmam/100
        % Over the maximum unbalance acceptance
        if Iarm > 0
            % charge the capacitors with lowest voltages
            Ons_next(order(Nb-N+1: Nb)) = ~Ons_next(order(Nb-N+1: Nb));
        else
            % discharge the capacitors with highest voltages
            Ons_next(order(1: N)) = ~Ons_next(order(1: N));
        end

    else
        if N-sum(Ons) ==  0
            % if we don't need to change the number of SM that is on
            Ons_next = Ons;
        
        elseif N-sum(Ons) > 0
            % if we need more SMs are to be on-state

            % number of SMs that needed to be changed the state
            DeltaN = N-sum(Ons);
            % keep previously being on SMs still being on
            Ons_next = Ons;

            if Iarm > 0
                % charge the capacitors with lowest voltages
                for i = 1: Nb
                    if DeltaN <= 0
                        break;
                    end
                    % if the SM is off and still need more SM
                    if Ons(order(Nb-i+1)) == false
                        DeltaN = DeltaN - 1;
                        Ons_next(order(Nb-i+1)) = true;
                    end
                end

            else
                % discharge the capacitors with highest voltages
                for i = 1: Nb
                    if DeltaN <= 0
                        break;
                    end
                    % if the SM is off and still need more SM
                    if Ons(order(i)) == false
                        DeltaN = DeltaN - 1;
                        Ons_next(order(i)) = true;
                    end
                end
            end

        else
            % if we need less SMs are to be on-state

            % number of SMs that needed to be changed the state
            DeltaN = sum(Ons)-N;
            % keep previously being on SMs still being on
            Ons_next = Ons;

            if Iarm > 0
                % remove the capacitor with highest voltage
                for i = 1: Nb
                    if DeltaN <= 0
                        break;
                    end
                    % if the SM is on and still need less SM
                    if Ons(order(i)) == true
                        DeltaN = DeltaN - 1;
                        Ons_next(order(i)) = false;
                    end
                end

            else
                % remove the capacitor with lowest voltage
                for i = 1: Nb
                    if DeltaN <= 0
                        break;
                    end
                    % if the SM is on and still need less SM
                    if Ons(order(Nb-i+1)) == true
                        DeltaN = DeltaN - 1;
                        Ons_next(order(Nb-i+1)) = false;
                    end
                end
            end
        end
    end
end

== matlab function Mmc/MMC/modulation/Sorting nb/MATLAB Function1 ==
  data: u input; y output
function y = FiringSorting(u)
    y = u;
    for i = 1: length(u)
        if mod(i, 2) == 1
            y(i) = u(int16(i/2));
        else
            y(i) = u(int16(i/2+length(u)/2));
        end
    end
end

== matlab function Mmc/MMC/modulation/Sorting pc/MATLAB Function ==
  data: Usm input; N input; Ons_next output; Sigmam input; Iarm input; Ons input
function Ons_next = SmFiringSorting(Usm, N, Sigmam, Iarm, Ons)
    %%%
    % SmFiringSorting -- SM firing sorting. -- C.SI on 5th, Oct.
    %% Inputs:
    % Usm - capacitor voltage on each SM;
    % N - number of SMs that needed to fire up;
    % Sigmam [%] - Maximum allowed voltage unbalance rate;
    % Iarm - arm current;
    % Ons (boolean) - indicate those SM(s) who are in series with the
    % source in the last control period;
    %% Outputs:
    % Ons_now (boolean) - indicate those SM(s) who should be in series with 
    % the source in this control period;
    %%%
    
    % number of SMs
    Nb = length(Usm);
    % initialize the on-state boolean array
    Ons_next = zeros(Nb, 1); 
    % rank the SMs in the order of descendance
    [~, order] = sort(Usm, 'descend');
    
    if max(abs(1-Usm)) > Sigmam/100
        % Over the maximum unbalance acceptance
        if Iarm > 0
            % charge the capacitors with lowest voltages
            Ons_next(order(Nb-N+1: Nb)) = ~Ons_next(order(Nb-N+1: Nb));
        else
            % discharge the capacitors with highest voltages
            Ons_next(order(1: N)) = ~Ons_next(order(1: N));
        end

    else
        if N-sum(Ons) ==  0
            % if we don't need to change the number of SM that is on
            Ons_next = Ons;
        
        elseif N-sum(Ons) > 0
            % if we need more SMs are to be on-state

            % number of SMs that needed to be changed the state
            DeltaN = N-sum(Ons);
            % keep previously being on SMs still being on
            Ons_next = Ons;

            if Iarm > 0
                % charge the capacitors with lowest voltages
                for i = 1: Nb
                    if DeltaN <= 0
                        break;
                    end
                    % if the SM is off and still need more SM
                    if Ons(order(Nb-i+1)) == false
                        DeltaN = DeltaN - 1;
                        Ons_next(order(Nb-i+1)) = true;
                    end
                end

            else
                % discharge the capacitors with highest voltages
                for i = 1: Nb
                    if DeltaN <= 0
                        break;
                    end
                    % if the SM is off and still need more SM
                    if Ons(order(i)) == false
                        DeltaN = DeltaN - 1;
                        Ons_next(order(i)) = true;
                    end
                end
            end

        else
            % if we need less SMs are to be on-state

            % number of SMs that needed to be changed the state
            DeltaN = sum(Ons)-N;
            % keep previously being on SMs still being on
            Ons_next = Ons;

            if Iarm > 0
                % remove the capacitor with highest voltage
                for i = 1: Nb
                    if DeltaN <= 0
                        break;
                    end
                    % if the SM is on and still need less SM
                    if Ons(order(i)) == true
                        DeltaN = DeltaN - 1;
                        Ons_next(order(i)) = false;
                    end
                end

            else
                % remove the capacitor with lowest voltage
                for i = 1: Nb
                    if DeltaN <= 0
                        break;
                    end
                    % if the SM is on and still need less SM
                    if Ons(order(Nb-i+1)) == true
                        DeltaN = DeltaN - 1;
                        Ons_next(order(Nb-i+1)) = false;
                    end
                end
            end
        end
    end
end

== matlab function Mmc/MMC/modulation/Sorting pc/MATLAB Function1 ==
  data: u input; y output
function y = FiringSorting(u)
    y = u;
    for i = 1: length(u)
        if mod(i, 2) == 1
            y(i) = u(int16(i/2));
        else
            y(i) = u(int16(i/2+length(u)/2));
        end
    end
end

== matlab function Mmc/MMC/modulation/Nearest Level Pulse Generator a /MATLAB Function ==
  data: u input; y output
function y = FiringSorting(u)
    y = u;
    for i = 1: length(u)
        if mod(i, 2) == 1
            y(i) = u(int16(i/2));
        else
            y(i) = u(int16(i/2+length(u)/2));
        end
    end
end
